simulink model "moteur_seul_22_09_2025"  (R2025a)
settings: Solver=VariableStepAuto  StartTime=0.0  StopTime=0.1  FixedStep=1e-4  RelTol=1e-3
undefined symbols (not defined in the file): J, Kphi, L, R, U
settings Model: Creator=ltroullier01  LastModifiedBy=ltroullier01

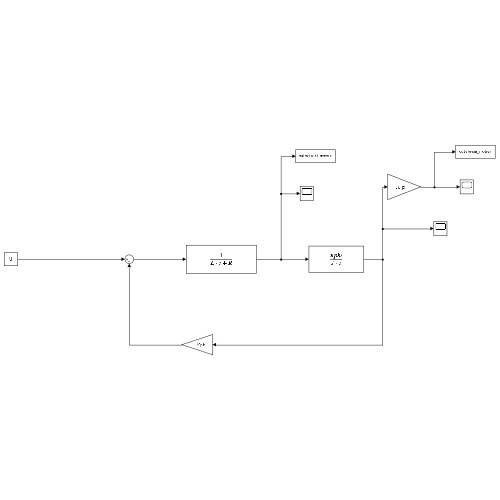
[thumbnail: Simulink's stored preview of the top-level diagram]
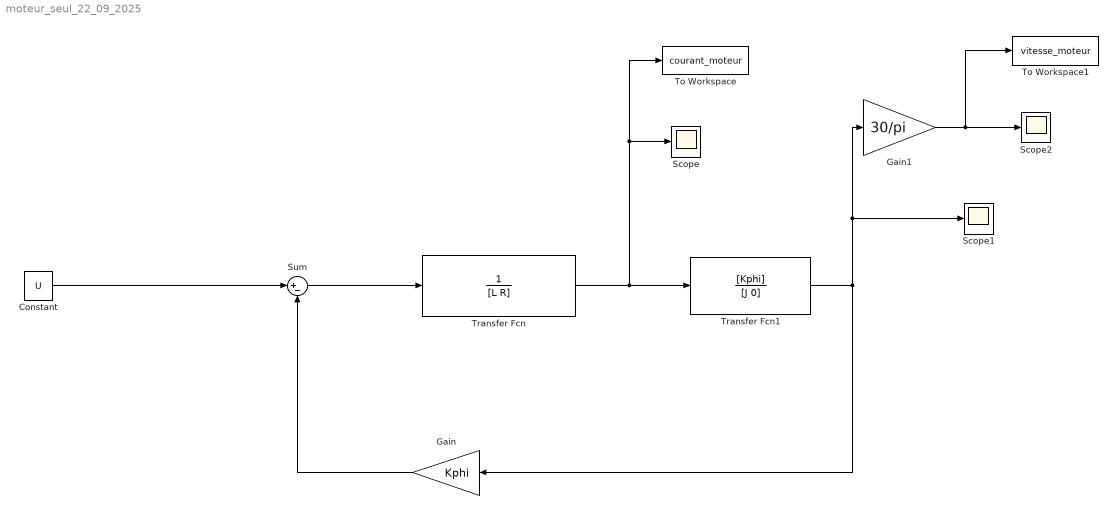
== system moteur_seul_22_09_2025 ==
  Constant : Constant  Value=U
  Gain : Gain  Gain=Kphi
  Gain1 : Gain  Gain=30/pi
  Scope : Scope
      settings: ActiveDisplayYMinimum=-4.9369832712561159  ActiveDisplayYMaximum=31.373841687864346
  Scope1 : Scope
      settings: ActiveDisplayYMinimum=-47.244091400346811  ActiveDisplayYMaximum=425.19682260312135
  Scope2 : Scope
      settings: ActiveDisplayYMinimum=-1903.7496929081253  ActiveDisplayYMaximum=5096.5030674299223  DataLoggingVariableName=ScopeData2
  Sum : Sum  Inputs=|+-
  To Workspace : ToWorkspace  VariableName=courant_moteur  SaveFormat=Timeseries  SampleTime=-1
  To Workspace1 : ToWorkspace  VariableName=vitesse_moteur  SaveFormat=Timeseries  SampleTime=-1
  Transfer Fcn : TransferFcn  Denominator=[L R]
  Transfer Fcn1 : TransferFcn  Numerator=[Kphi]  Denominator=[J 0]
  wires:
  Constant/1 -> Sum/1
  Sum/1 -> Transfer Fcn/1
  Transfer Fcn/1 -> To Workspace/1, Scope/1, Transfer Fcn1/1
  Transfer Fcn1/1 -> Scope1/1, Gain1/1, Gain/1
  Gain/1 -> Sum/2
  Gain1/1 -> To Workspace1/1, Scope2/1
